simulink model "weightmodel"  (R2019a)
settings: Solver=FixedStepAuto  StartTime=0.0  StopTime=20  FixedStep=Ts  RelTol=1e-3  EnableMultiTasking=on
values from neighbouring files (symbols this model uses):
  f1_off = 0    [msstudy.m]    (also in pbase_l.m = nanmean(tsmovavg(Input3.data(1:40000,1),'s',1000,1)))
  f2_off = 0    [msstudy.m]    (also in pbase_l.m = nanmean(tsmovavg(Input3.data(1:40000,2),'s',1000,1)))
  f3_off = 0    [msstudy.m]    (also in pbase_l.m = nanmean(tsmovavg(Input3.data(1:40000,3),'s',1000,1)))
  f4_off = 0    [msstudy.m]    (also in pbase_l.m = nanmean(tsmovavg(Input3.data(1:40000,4),'s',1000,1)))
  f5_off = 0    [msstudy.m]    (also in pbase_l.m = nanmean(tsmovavg(Input3.data(1:40000,5),'s',1000,1)))
  f6_off = 0    [msstudy.m]    (also in pbase_l.m = nanmean(tsmovavg(Input3.data(1:40000,6),'s',1000,1)))
  Ts = 0.0005    [msstudy.m]
undefined symbols (not defined in the file or in its folder): Pull, up
libraries: speedgoatlib_IO183 x4, slrtlib x2
settings Model: Creator=vnalam  LastModifiedBy=vnalam
settings DataIOCC: LimitDataPoints=on  SaveFormat=StructureWithTime  ReturnWorkspaceOutputs=off
settings OptimizationCC: BlockReduction=off  OptimizeBlockIOStorage=off  BufferReuse=off  GlobalBufferReuse=off  ExpressionFolding=off  LocalBlockOutputs=off  LifeSpan=inf  OptimizeDataStoreBuffers=off  BusAssignmentInplaceUpdate=off
settings DebuggingCC: AllowSymbolicDim=off  SFUnexpectedBacktrackingDiag=warning  SFNoUnconditionalDefaultTransitionDiag=warning  SFExecutionAtInitializationDiag=none  ArithmeticOperatorsInVariantConditions=warning
settings HardwareCC: ProdBitPerPointer=32  ProdBitPerSizeT=32  ProdBitPerPtrDiffT=32  ProdLargestAtomicFloat=None  ProdWordSize=32  ProdLongLongMode=on  ProdHWDeviceType=Generic->32-bit x86 compatible
settings ModelReferenceCC: PropagateSignalLabelsOutOfModel=off
settings SFSimCC: SimUseLocalCustomCode=off
settings RTWCC: SystemTargetFile=slrt.tlc  TLCOptions=-axPCModelStackSizeKB=512  TemplateMakefile=slrt_default_tmf  Description=Simulink Real-Time  RTWUseLocalCustomCode=off  CodeExecutionProfiling=on  RTWCompilerOptimization=on
settings CodeAppCC: StateflowObjectComments=on
settings SimulinkRealTimeCC: PreserveStateflowLocalDataDimensions=off  xPCisDownloadable=off
settings ConfigComp: CovMetricSettings=dw  CovHtmlReporting=on  CovSaveCumulativeToWorkspaceVar=on  CovSaveSingleToWorkspaceVar=on  CovExternalEMLEnable=off

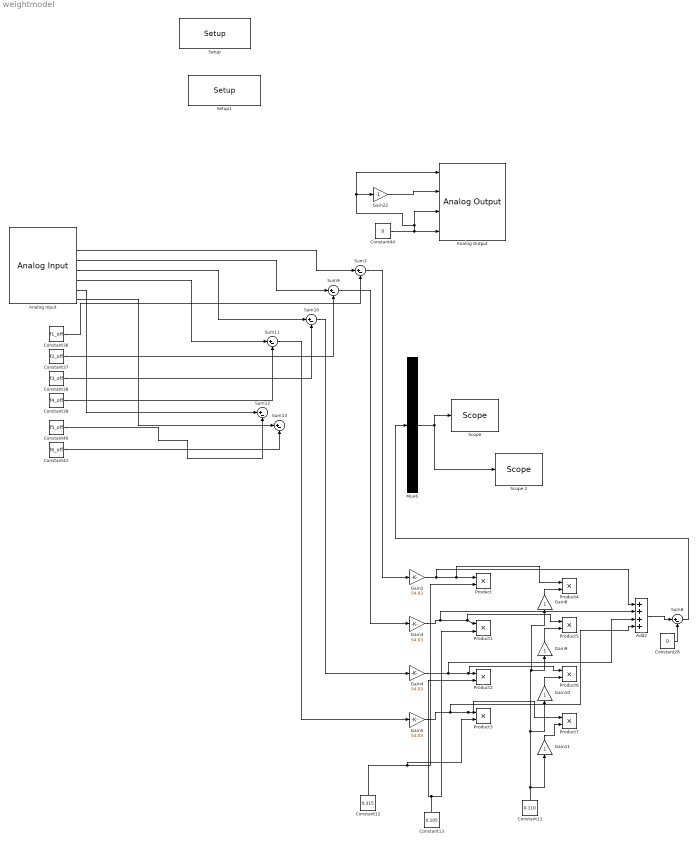
== system weightmodel ==
  Add2 : Sum  Inputs=++++
  Analog Input : speedgoatlib_IO183/Analog Input  Priority=0  parModuleId=1  parSampTime=Ts  parPciSlot=-1  parAdChannelLow=1  parAdChannelHigh=8
      settings: SourceProductName=Simulink Real-Time: Speedgoat Library
  Analog Output : speedgoatlib_IO183/Analog Output  parModuleId=1  parSampTime=Ts  parDaSimult=on  parPciSlot=-1  parDaChannels=[1 2 3 4]  parDaInit=[0 0 0 0]  parDaReset=[0 0 0 0]
      settings: SourceProductName=Simulink Real-Time: Speedgoat Library
  Constant11 : Constant  Value=0.110  SampleTime=-1
  Constant12 : Constant  Value=0.315  SampleTime=-1
  Constant13 : Constant  Value=0.105  SampleTime=-1
  Constant28 : Constant  Value=0  SampleTime=Ts
  Constant36 : Constant  Value=f1_off  SampleTime=Ts
  Constant37 : Constant  Value=f2_off  SampleTime=Ts
  Constant38 : Constant  Value=f3_off  SampleTime=Ts
  Constant39 : Constant  Value=f4_off  SampleTime=Ts
  Constant40 : Constant  Value=f5_off  SampleTime=Ts
  Constant41 : Constant  Value=f6_off  SampleTime=Ts
  Constant44 : Constant  Value=0  SampleTime=Ts
  Gain{8..11} (4 alike) : Gain
  Gain{2..5} (4 alike) : Gain  Gain=54.03
  Gain22 : Gain  Gain=-1
  Mux6 : Mux  Inputs=1
  Product{,1..7} (8 alike) : Product
  "Scope " : slrtlib/Displays and Logging/Scope   scopeno=3  scopetype=File  autostart=on  viewmode=Graphical redraw  formatstr='%15.6f'  grid=on  ylimits=[0,0]  nosamples=800000  noprepostsamples=0  interleave=1  triggermode=FreeRun  triggersignal=1  trigsignalfromport=off  triggerlevel=0.0  triggerslope=Either  triggerscope=1  triggersample=0  filename=weight.dat  mode=Lazy  writesize=512  autorestart=off  dynamicfilemode=off  maxwritefilesize=512*1024^2
  Scope 2 : slrtlib/Displays and Logging/Scope   scopeno=2  scopetype=Target  autostart=on  viewmode=Graphical rolling  formatstr='%15.6f'  grid=on  ylimits=[0,0]  nosamples=40000  noprepostsamples=0  interleave=1  triggermode=FreeRun  triggersignal=1  trigsignalfromport=off  triggerlevel=0.0  triggerslope=Either  triggerscope=1  triggersample=0  filename=tot303.dat  mode=Lazy  writesize=512  autorestart=off  dynamicfilemode=off  maxwritefilesize=512*1024^2
  Setup : speedgoatlib_IO183/Setup  parModuleId=1  parPciSlot=-1  parDaSimult=on  parAdCoupling=Single Ended  parAdRange=+-10V  parAdChannelLow=1  parAdChannelHigh=8  parDaChannels=[1:4]  parDaRange=0..5V  parDaInit=[0]  parDaReset=[0]  parDoChannels=[1:8]  parDoInit=[0]  parDoReset=[1]  parDiChannels=[9:16]  parIOPullReferenceFront=Pull-up (3.3V)  parIOPullReferenceRear=Pull-up (3.3V)
      settings: SourceProductName=Simulink Real-Time: Speedgoat Library
  Setup1 : speedgoatlib_IO183/Setup  parModuleId=2  parPciSlot=-1  parDaSimult=on  parAdCoupling=Single Ended  parAdRange=+-10V  parAdChannelLow=1  parAdChannelHigh=8  parDaChannels=[1:4]  parDaRange=0..5V  parDaInit=[0]  parDaReset=[0]  parDoChannels=[1:8]  parDoInit=[0]  parDoReset=[1]  parDiChannels=[9:16]  parIOPullReferenceFront=Pull-up (3.3V)  parIOPullReferenceRear=Pull-up (3.3V)
      settings: SourceProductName=Simulink Real-Time: Speedgoat Library
  Sum{3,8..13} (7 alike) : Sum  Inputs=|+-
  wires:
  Gain2/1 -> Add2/1, Product4/1, Product/1
  Gain3/1 -> Add2/2, Product5/1, Product1/1
  Gain4/1 -> Add2/3, Product6/1, Product2/1
  Gain5/1 -> Add2/4, Product7/1, Product3/1
  Constant11/1 -> Gain8/1, Gain9/1, Gain10/1, Gain11/1
  Gain8/1 -> Product4/2
  Gain9/1 -> Product5/2
  Gain10/1 -> Product6/2
  Gain11/1 -> Product7/2
  Constant13/1 -> Product2/2, Product1/2
  Constant12/1 -> Product3/2, Product/2
  Constant44/1 -> Analog Output/4, Analog Output/1, Gain22/1, Analog Output/3
  Sum9/1 -> Gain3/1
  Sum10/1 -> Gain4/1
  Sum11/1 -> Gain5/1
  Sum3/1 -> Gain2/1
  Constant28/1 -> Sum8/2
  Add2/1 -> Sum8/1
  Analog Input/3 -> Sum3/1
  Analog Input/5 -> Sum10/1
  Analog Input/4 -> Sum9/1
  Analog Input/6 -> Sum11/1
  Constant36/1 -> Sum3/2
  Constant37/1 -> Sum9/2
  Constant38/1 -> Sum10/2
  Constant39/1 -> Sum11/2
  Analog Input/7 -> Sum12/1
  Constant40/1 -> Sum12/2
  Analog Input/8 -> Sum13/1
  Constant41/1 -> Sum13/2
  Gain22/1 -> Analog Output/2
  Sum8/1 -> Mux6/1
  Mux6/1 -> "Scope "/1, Scope 2/1
